simulink model "gm_uz_deadbeat_clean"  (R2022a)
settings: Solver=FixedStepDiscrete  StartTime=0.0  StopTime=1  RelTol=1e-3
libraries: hdlmdlgenlib x120, spsCurrentMeasurementLib x3, spsSeriesRLCBranchLib x2, spsDCVoltageSourceLib x1, spsPWMGenerator2LevelLib x1, spsPermanentMagnetSynchronousMachineLib x1, spsTwoLevelConverterLib x1, spsabctodq0Lib x1, spspowerguiLib x1
settings Model: Creator=go98noz  LastModifiedBy=go98noz
settings SolverCC: AlgebraicLoopSolver=TrustRegion  AutoInsertRateTranBlk=on
settings DataIOCC: LimitDataPoints=on  SaveOutput=off  SaveTime=off
settings OptimizationCC: BlockReduction=off  ConditionallyExecuteInputs=off  DefaultParameterBehavior=Inlined  InheritOutputTypeSmallerThanSingle=on  LifeSpan=inf
settings DebuggingCC: AlgebraicLoopMsg=error  InheritedTsInSrcMsg=none  SingleTaskRateTransMsg=error  UnconnectedInputMsg=warning  UnconnectedOutputMsg=warning  UnconnectedLineMsg=warning  AllowSymbolicDim=off  StrictBusMsg=ErrorOnBusTreatedAsVector  SFUnexpectedBacktrackingDiag=warning  SFNoUnconditionalDefaultTransitionDiag=warning  SFExecutionAtInitializationDiag=none  SFMachineParentedDataDiag=warning  ArithmeticOperatorsInVariantConditions=warning
settings HardwareCC: ProdBitPerPointer=32  ProdBitPerSizeT=32  ProdBitPerPtrDiffT=32  ProdLargestAtomicFloat=None  ProdIntDivRoundTo=Undefined  ProdEndianess=Unspecified  ProdWordSize=32  ProdHWDeviceType=ASIC/FPGA->ASIC/FPGA  ProdEqTarget=off
settings SFSimCC: SimUseLocalCustomCode=off  CustomCodeUndefinedFunction=UseInterfaceOnly
settings RTWCC: RTWUseLocalCustomCode=off
settings CodeAppCC: StateflowObjectComments=on
settings GRTTargetCC: TargetLangStandard=C89/C90 (ANSI)
settings ConfigComp: CovScope=ReferencedModels  CovMetricSettings=dw  CovSaveCumulativeToWorkspaceVar=on  CovSaveSingleToWorkspaceVar=on  CovExternalEMLEnable=off  CovSFcnEnable=off

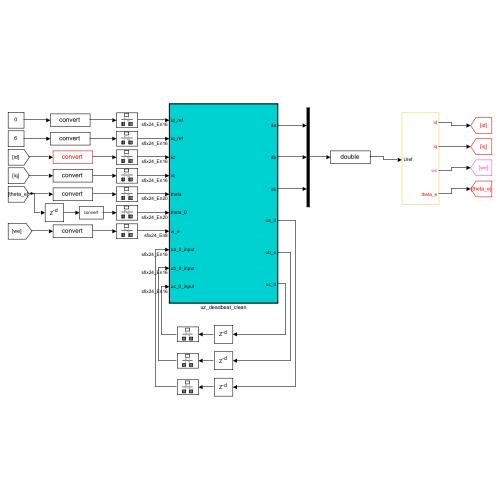
[thumbnail: Simulink's stored preview of the top-level diagram]
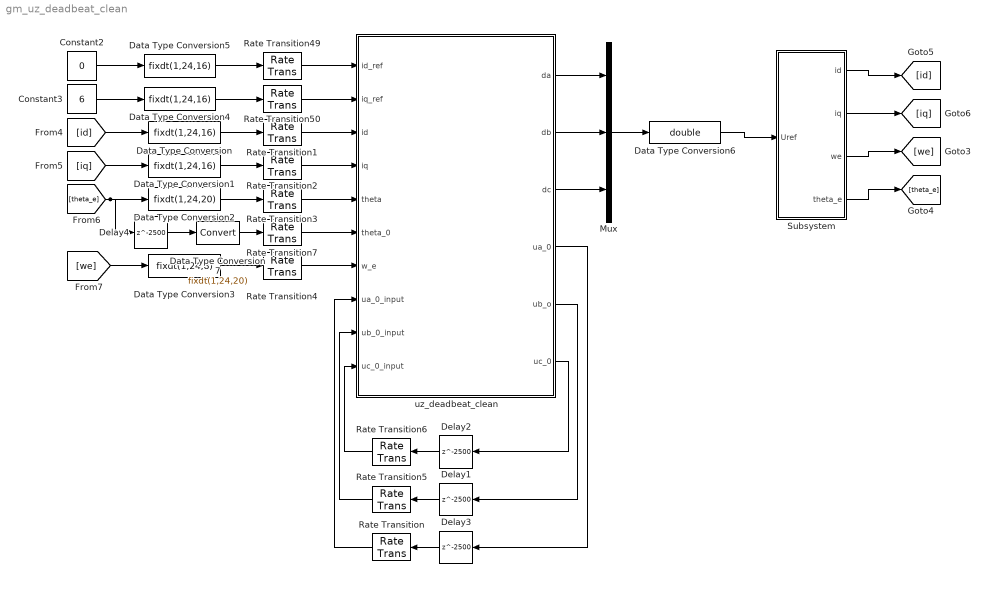
== system gm_uz_deadbeat_clean ==
  Constant2 : Constant  Value=0
  Constant3 : Constant  Value=6
  Data Type Conversion{,1,4..5} (4 alike) : DataTypeConversion  OutDataTypeStr=fixdt(1,24,16)  SaturateOnIntegerOverflow=off  RndMeth=Floor
  Data Type Conversion2 : DataTypeConversion  OutDataTypeStr=fixdt(1,24,20)  SaturateOnIntegerOverflow=off  RndMeth=Floor
  Data Type Conversion3 : DataTypeConversion  OutDataTypeStr=fixdt(1,24,8)  SaturateOnIntegerOverflow=off  RndMeth=Floor
  Data Type Conversion6 : DataTypeConversion  OutDataTypeStr=double  SaturateOnIntegerOverflow=off  RndMeth=Floor
  Data Type Conversion7 : DataTypeConversion  OutDataTypeStr=fixdt(1,24,20)  SaturateOnIntegerOverflow=off  RndMeth=Floor
  Delay{1..4} (4 alike) : Delay  DelayLength=2500  SampleTime=1e-8
  Mux : Mux  Inputs=3
  Rate Transition{,1..7,49..50} (10 alike) : RateTransition  OutPortSampleTime=1e-8
  Subsystem : Subsystem
  uz_deadbeat_clean : Subsystem  TreatAsAtomicUnit=on
  wires:
  Data Type Conversion7/1 -> Rate Transition7/1
  Rate Transition7/1 -> uz_deadbeat_clean/6(theta_0)
  Delay4/1 -> Data Type Conversion7/1
  Rate Transition/1 -> uz_deadbeat_clean/8(ua_0_input)
  Rate Transition6/1 -> uz_deadbeat_clean/10(uc_0_input)
  Rate Transition5/1 -> uz_deadbeat_clean/9(ub_0_input)
  uz_deadbeat_clean/6(uc_0) -> Delay2/1
  Delay2/1 -> Rate Transition6/1
  Delay1/1 -> Rate Transition5/1
  uz_deadbeat_clean/5(ub_o) -> Delay1/1
  Delay3/1 -> Rate Transition/1
  uz_deadbeat_clean/4(ua_0) -> Delay3/1
  Subsystem/4(theta_e) -> [theta_e]
  Subsystem/3(we) -> [we]
  Subsystem/2(iq) -> [iq]
  Subsystem/1(id) -> [id]
  Data Type Conversion6/1 -> Subsystem/1(Uref)
  uz_deadbeat_clean/3(dc) -> Mux/3
  uz_deadbeat_clean/2(db) -> Mux/2
  uz_deadbeat_clean/1(da) -> Mux/1
  Rate Transition4/1 -> uz_deadbeat_clean/7(w_e)
  [we] -> Data Type Conversion3/1
  Rate Transition3/1 -> uz_deadbeat_clean/5(theta)
  [theta_e] -> Data Type Conversion2/1, Delay4/1
  Rate Transition2/1 -> uz_deadbeat_clean/4(iq)
  [iq] -> Data Type Conversion1/1
  Rate Transition1/1 -> uz_deadbeat_clean/3(id)
  [id] -> Data Type Conversion/1
  Rate Transition50/1 -> uz_deadbeat_clean/2(iq_ref)
  Constant3/1 -> Data Type Conversion4/1
  Constant2/1 -> Data Type Conversion5/1
  Data Type Conversion2/1 -> Rate Transition3/1
  Data Type Conversion5/1 -> Rate Transition49/1
  Data Type Conversion/1 -> Rate Transition1/1
  Data Type Conversion4/1 -> Rate Transition50/1
  Data Type Conversion3/1 -> Rate Transition4/1
  Data Type Conversion1/1 -> Rate Transition2/1
  Rate Transition49/1 -> uz_deadbeat_clean/1(id_ref)
  Mux/1 -> Data Type Conversion6/1

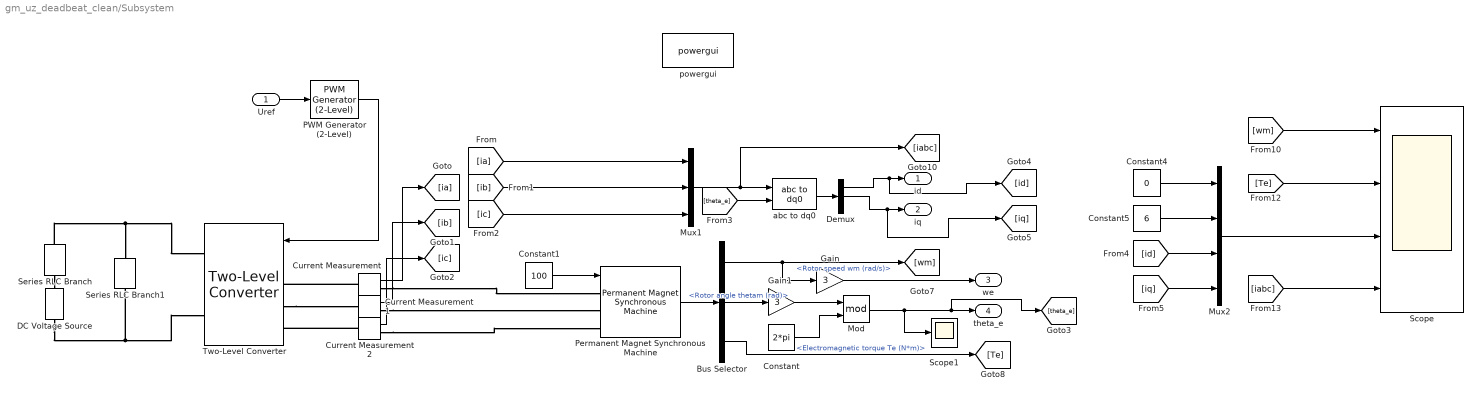
== system gm_uz_deadbeat_clean/Subsystem ==
  Uref : Inport
  Bus Selector : BusSelector  OutputSignals=Rotor speed wm (rad/s),Rotor angle thetam (rad),Electromagnetic torque Te (N*m)
  Constant : Constant  Value=2*pi
  Constant1 : Constant  Value=100
  Constant4 : Constant  Value=0
  Constant5 : Constant  Value=6
  Current Measurement : spsCurrentMeasurementLib/Current Measurement  PhasorSimulation=off  OutputType=Complex  PSBequivalent=0
  Current Measurement1 : spsCurrentMeasurementLib/Current Measurement  PhasorSimulation=off  OutputType=Complex  PSBequivalent=0
  Current Measurement2 : spsCurrentMeasurementLib/Current Measurement  PhasorSimulation=off  OutputType=Complex  PSBequivalent=0
  DC Voltage Source : spsDCVoltageSourceLib/DC Voltage Source  Amplitude=340  Measurements=None
  Demux : Demux  Outputs=3
  Gain : Gain  Gain=3
  Gain1 : Gain  Gain=3
  Mod : Math  Operator=mod
  Mux1 : Mux  Inputs=3
  Mux2 : Mux
  PWM Generator (2-Level) : spsPWMGenerator2LevelLib/PWM Generator (2-Level)  ModulatorType=Three-phase bridge (6 pulses)  ModulatorMode=Unsynchronized  Fc=20e3  Pc=0  nF=27  MinMax="[ 0  1 ]"  SamplingTechnique=Asymmetrical regular (double edge)  ModulatingSignals=off  m=0.8  Freq=60  Phase=0  Ts=1e-8  ShowCarrierOutport=off
  Permanent Magnet Synchronous Machine : spsPermanentMagnetSynchronousMachineLib/Permanent Magnet Synchronous Machine  NbPhases=3  FluxDistribution=Sinusoidal  RotorType=Round  MechanicalLoad=Speed w  PresetModel=No  ShowDetailedParameters=on  MeasurementBus=off  Resistance=1.2  Inductance=8.5e-3  dqInductances=[8.5e-3,8.5e-3]  La=0.0136  MachineConstant=Flux linkage established by magnets (V.s)  Flux=0.140  VoltageCst=76.1796  TorqueCst=0.63  Flat=120  Mechanical=[0.0002506 0.0004924 3 0]  PolePairs=3  InitialConditions=[100,0, 0,0]  InitialConditions5ph=[0 0 0 0 0 0]  RefAngle=Aligned with phase A axis (original Park)  IterativeDiscreteModel=Trapezoidal non iterative  TsBlock=-1  TsPowergui=0
  Scope : Scope  NumInputPorts=4
  Scope1 : Scope
  Series RLC Branch : spsSeriesRLCBranchLib/Series RLC Branch  LConnTagsString=__new0  RConnTagsString=__new0  BranchType=R  Resistance=1e-3  Inductance=1e-3  SetiL0=off  InitialCurrent=0  Capacitance=1e-6  Setx0=off  InitialVoltage=0  Measurements=None
  Series RLC Branch1 : spsSeriesRLCBranchLib/Series RLC Branch  LConnTagsString=__new0  RConnTagsString=__new0  BranchType=C  Resistance=1e-3  Inductance=1e-3  SetiL0=off  InitialCurrent=0  Capacitance=3300e-6  Setx0=off  InitialVoltage=0  Measurements=None
  Two-Level Converter : spsTwoLevelConverterLib/Two-Level Converter  ModelType=Switching devices  Ron=1e-3  Rs=1e6  Cs=inf  Vforward=[0,0]  Ron_Diode=1e-3  Rs_Diode=1e6  Cs_Diode=inf  Vf_Diode=1e-3  Rs_CurrentSource=inf  Ron_ACsource=1e-3
      settings: SourceProductBaseCode=PS
  abc to dq0 : spsabctodq0Lib/abc to dq0  Alignment=Aligned with phase A axis
  powergui : spspowerguiLib/powergui  Priority=1  SimulationMode=Discrete  SampleTime=1e-8  frequency=60  Iterations=50  frequencyindice=0  Pbase=100e6  ErrMax=1e-4  UnitsV=kV  UnitsW=MW  buscounter=0  FunctionMessages=off  echomessages=off  EnableUseOfTLC=off  CurrentSourceSwitches=off  DisableSnubberDevices=off  DisableRonSwitches=off  DisableVfSwitches=off  DisplayEquations=off  AutomaticDiscreteSolvers=off  SolverType=Tustin/Backward Euler (TBE)  Interpol=off  ExternalGateDelay=off  methode=off  Ts=100  x0status=blocks  SPID=on  SwTol=0  HookPort=off  NonlinearTolerance=1e-4  nMaxIteration=100  ContinueOnMaxIteration=off  RestoreLinks=warning  ResistiveCurrentMeasurement=off  Frange=[0:2:500]  Ylog=off  Xlog=on  ShowGrid=off  save=off  variable=ZData  structure=0  ZoomFFT=off  StartTime=0.0  cycles=1  DisplayStyle=1  fundamental=60  FreqAxis=off  MaxFrequency=1000  frequencyindicesteady=1  RmsSteady=1  display=off
  id : Outport
  iq : Outport  Port=2
  we : Outport  Port=3
  theta_e : Outport  Port=4
  wires:
  [ib] -> Mux1/2
  Bus Selector/3 -> [Te]  "<Electromagnetic torque Te (N*m)>"
  abc to dq0/1 -> Demux/1
  Current Measurement1/1 -> [ib]
  [wm] -> Scope/1
  [iabc] -> Scope/4
  [ia] -> Mux1/1
  [id] -> Mux2/3
  [Te] -> Scope/2
  Current Measurement/1 -> [ia]
  Constant4/1 -> Mux2/1
  Mod/1 -> Scope1/1, theta_e/1, [theta_e]
  Uref/1 -> PWM Generator (2-Level)/1
  Permanent Magnet Synchronous Machine/1 -> Bus Selector/1
  Gain1/1 -> Mod/1
  [ic] -> Mux1/3
  Demux/2 -> iq/1, [iq]
  Demux/1 -> id/1, [id]
  Bus Selector/1 -> [wm], Gain/1  "<Rotor speed wm (rad/s)>"
  Bus Selector/2 -> Gain1/1  "<Rotor angle thetam (rad)>"
  [theta_e] -> abc to dq0/2
  Mux1/1 -> abc to dq0/1, [iabc]
  Gain/1 -> we/1
  Mux2/1 -> Scope/3
  Constant5/1 -> Mux2/2
  [iq] -> Mux2/4
  Current Measurement2/1 -> [ic]
  Constant1/1 -> Permanent Magnet Synchronous Machine/1
  PWM Generator (2-Level)/1 -> Two-Level Converter/1
  Constant/1 -> Mod/2
  connections:
  Current Measurement/RConn1 -- Permanent Magnet Synchronous Machine/LConn1
  Current Measurement2/LConn1 -- Two-Level Converter/LConn3
  Two-Level Converter/LConn2 -- Current Measurement1/LConn1
  Series RLC Branch/LConn1 -- Series RLC Branch1/LConn1 -- Two-Level Converter/RConn1
  Current Measurement1/RConn1 -- Permanent Magnet Synchronous Machine/LConn2
  Series RLC Branch/RConn1 -- DC Voltage Source/RConn1
  Current Measurement2/RConn1 -- Permanent Magnet Synchronous Machine/LConn3
  Current Measurement/LConn1 -- Two-Level Converter/LConn1
  DC Voltage Source/LConn1 -- Two-Level Converter/RConn2 -- Series RLC Branch1/RConn1

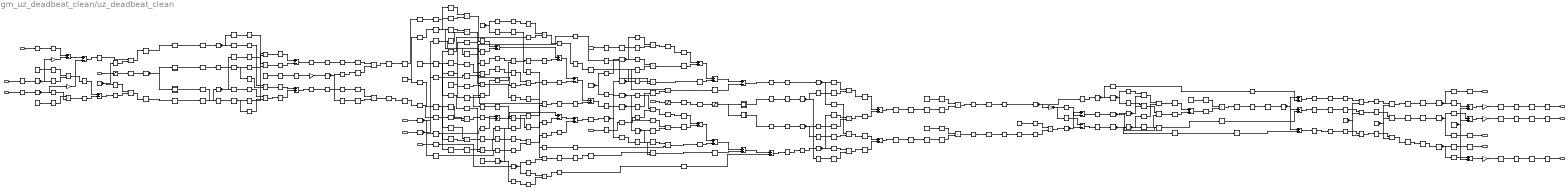
== system gm_uz_deadbeat_clean/uz_deadbeat_clean ==
  id_ref : Inport  OutDataTypeStr=fixdt(1, 24, 16)  PortDimensions=1  SampleTime=1e-08
  iq_ref : Inport  Port=2  OutDataTypeStr=fixdt(1, 24, 16)  PortDimensions=1  SampleTime=1e-08
  id : Inport  Port=3  OutDataTypeStr=fixdt(1, 24, 16)  PortDimensions=1  SampleTime=1e-08
  iq : Inport  Port=4  OutDataTypeStr=fixdt(1, 24, 16)  PortDimensions=1  SampleTime=1e-08
  theta : Inport  Port=5  OutDataTypeStr=fixdt(1, 24, 20)  PortDimensions=1  SampleTime=1e-08
  theta_0 : Inport  Port=6  OutDataTypeStr=fixdt(1, 24, 20)  PortDimensions=1  SampleTime=1e-08
  w_e : Inport  Port=7  OutDataTypeStr=fixdt(1, 24, 8)  PortDimensions=1  SampleTime=1e-08
  ua_0_input : Inport  Port=8  OutDataTypeStr=fixdt(1, 24, 16)  PortDimensions=1  SampleTime=1e-08
  ub_0_input : Inport  Port=9  OutDataTypeStr=fixdt(1, 24, 16)  PortDimensions=1  SampleTime=1e-08
  uc_0_input : Inport  Port=10  OutDataTypeStr=fixdt(1, 24, 16)  PortDimensions=1  SampleTime=1e-08
  Add1 : Sum  Inputs=+-  AccumDataTypeStr=fixdt(1, 49, 39)  OutDataTypeStr=fixdt(1, 49, 39)  SampleTime=1e-08
  Add10 : Sum  Inputs=+-  AccumDataTypeStr=fixdt(1, 49, 24)  OutDataTypeStr=fixdt(1, 49, 24)  SampleTime=1e-08
  Add11 : Sum  AccumDataTypeStr=fixdt(1, 49, 24)  OutDataTypeStr=fixdt(1, 49, 24)  SampleTime=1e-08
  Add12 : Sum  Inputs=+-  AccumDataTypeStr=fixdt(1, 49, 39)  OutDataTypeStr=fixdt(1, 49, 39)  SampleTime=1e-08
  Add13 : Sum  Inputs=--  AccumDataTypeStr=fixdt(1, 50, 39)  OutDataTypeStr=fixdt(1, 50, 39)  SampleTime=1e-08
  Add{14..20} (7 alike) : Sum  AccumDataTypeStr=fixdt(1, 25, 16)  OutDataTypeStr=fixdt(1, 25, 16)  SampleTime=1e-08
  Add2 : Sum  AccumDataTypeStr=fixdt(1, 49, 32)  OutDataTypeStr=fixdt(1, 49, 32)  SampleTime=1e-08
  Add3 : Sum  Inputs=+-  AccumDataTypeStr=fixdt(1, 49, 32)  OutDataTypeStr=fixdt(1, 49, 32)  SampleTime=1e-08
  Add4_stage2 : Sum  AccumDataTypeStr=fixdt(1, 83, 56)  OutDataTypeStr=fixdt(1, 49, 30)  SampleTime=1e-08
  Add4_stage3 : Sum  Inputs=+-  AccumDataTypeStr=fixdt(1, 83, 56)  OutDataTypeStr=fixdt(1, 83, 56)  SampleTime=1e-08
  Add4_stage4 : Sum  AccumDataTypeStr=fixdt(1, 83, 56)  OutDataTypeStr=fixdt(1, 83, 56)  SampleTime=1e-08
  Add5_stage2 : Sum  AccumDataTypeStr=fixdt(1, 83, 56)  OutDataTypeStr=fixdt(1, 49, 30)  SampleTime=1e-08
  Add5_stage3 : Sum  Inputs=+-  AccumDataTypeStr=fixdt(1, 83, 56)  OutDataTypeStr=fixdt(1, 83, 56)  SampleTime=1e-08
  Add5_stage4 : Sum  Inputs=+-  AccumDataTypeStr=fixdt(1, 83, 56)  OutDataTypeStr=fixdt(1, 83, 56)  SampleTime=1e-08
  Add5_stage5 : Sum  Inputs=+-  AccumDataTypeStr=fixdt(1, 83, 56)  OutDataTypeStr=fixdt(1, 83, 56)  SampleTime=1e-08
  Add7_stage2 : Sum  Inputs=+-  AccumDataTypeStr=fixdt(1, 73, 44)  OutDataTypeStr=fixdt(1, 73, 44)  SampleTime=1e-08
  Add7_stage3 : Sum  AccumDataTypeStr=fixdt(1, 73, 44)  OutDataTypeStr=fixdt(1, 74, 44)  SampleTime=1e-08
  Add7_stage4 : Sum  Inputs=+-  AccumDataTypeStr=fixdt(1, 73, 44)  OutDataTypeStr=fixdt(1, 73, 44)  SampleTime=1e-08
  Add8_stage2 : Sum  Inputs=+-  AccumDataTypeStr=fixdt(1, 73, 44)  OutDataTypeStr=fixdt(1, 73, 44)  SampleTime=1e-08
  Add8_stage3 : Sum  AccumDataTypeStr=fixdt(1, 73, 44)  OutDataTypeStr=fixdt(1, 74, 44)  SampleTime=1e-08
  Add8_stage4 : Sum  AccumDataTypeStr=fixdt(1, 73, 44)  OutDataTypeStr=fixdt(1, 75, 44)  SampleTime=1e-08
  Add8_stage5 : Sum  AccumDataTypeStr=fixdt(1, 73, 44)  OutDataTypeStr=fixdt(1, 73, 44)  SampleTime=1e-08
  Add_stage2 : Sum  Inputs=+-  AccumDataTypeStr=fixdt(1, 50, 39)  OutDataTypeStr=fixdt(1, 50, 39)  SampleTime=1e-08
  Add_stage3 : Sum  Inputs=+-  AccumDataTypeStr=fixdt(1, 50, 39)  OutDataTypeStr=fixdt(1, 50, 39)  SampleTime=1e-08
  Constant : Constant  Value=0.6666717529296875  OutDataTypeStr=fixdt(1, 24, 16)  SampleTime=1e-08
  Constant1 : Constant  Value=2.50004231929779052734375e-05  OutDataTypeStr=fixdt(0, 32, 30)  SampleTime=1e-08
  Constant10 : Constant  Value=0.001838207244873046875  OutDataTypeStr=fixdt(0, 24, 22)  SampleTime=1e-08
  Constant12 : Constant  Value=544  OutDataTypeStr=fixdt(0, 24, 8)  SampleTime=1e-08
  Constant2 : Constant  Value=1.200000762939453125  OutDataTypeStr=fixdt(1, 24, 18)  SampleTime=1e-08
  Constant3 : Constant  Value=0.01360034942626953125  OutDataTypeStr=fixdt(0, 24, 20)  SampleTime=1e-08
  Constant5 : Constant  Value=0.1400001049041748046875  OutDataTypeStr=fixdt(0, 24, 22)  SampleTime=1e-08
  Constant6 : Constant  Value=340  OutDataTypeStr=fixdt(0, 24, 8)  SampleTime=1e-08
  Constant7 : Constant  Value=-1  OutDataTypeStr=fixdt(1, 24, 16)  SampleTime=1e-08
  Constant8 : Constant  OutDataTypeStr=fixdt(1, 24, 16)  SampleTime=1e-08
  Constant9 : Constant  OutDataTypeStr=fixdt(1, 24, 16)  SampleTime=1e-08
  Data Type Conversion{6..11,14..15,22..38} (25 alike) : DataTypeConversion  OutDataTypeStr=fixdt(1, 24, 16)  SampleTime=1e-08  SaturateOnIntegerOverflow=off  RndMeth=Floor
  Data Type Conversion{12..13,17..18,20..21} (6 alike) : DataTypeConversion  OutDataTypeStr=fixdt(1, 24, 8)  SampleTime=1e-08  SaturateOnIntegerOverflow=off  RndMeth=Floor
  Data Type Conversion48 : DataTypeConversion  OutDataTypeStr=fixdt(0, 24, 8)  SampleTime=1e-08  SaturateOnIntegerOverflow=off  RndMeth=Floor
  From{,1..21,24..30,36..41,44..50,54..60,62..80,82} (69 alike) : hdlmdlgenlib/Buffer
      settings: SourceProductBaseCode=SL
  From_outbuff_out_pipe : Delay  DelayLength=double(10)  InitialCondition=0  SampleTime=1e-08
  Gain : Product  Inputs=**  OutDataTypeStr=fixdt(1, 48, 38)  SampleTime=1e-08
  Gain1 : Gain  Gain="fi(0,1,24,23,\"hex\",\"400000\")"  ParamDataTypeStr=fixdt(1, 24, 23)  OutDataTypeStr=fixdt(1, 48, 39)  SampleTime=1e-08
  Gain10 : Gain  Gain="fi(0,1,25,24,\"hex\",\"0800000\")"  ParamDataTypeStr=fixdt(1, 25, 24)  OutDataTypeStr=fixdt(1, 50, 40)  SampleTime=1e-08
  Gain11 : Gain  Gain="fi(0,1,25,24,\"hex\",\"0800000\")"  ParamDataTypeStr=fixdt(1, 25, 24)  OutDataTypeStr=fixdt(1, 50, 40)  SampleTime=1e-08
  Gain12 : Product  Inputs=**  OutDataTypeStr=fixdt(1, 48, 38)  SampleTime=1e-08
  Gain12_const : Constant  Value=0.00588000006973743438720703125  OutDataTypeStr=fixdt(1, 24, 30)  SampleTime=1e-08
  Gain2 : Gain  Gain="fi(0,1,24,23,\"hex\",\"400000\")"  ParamDataTypeStr=fixdt(1, 24, 23)  OutDataTypeStr=fixdt(1, 48, 39)  SampleTime=1e-08
  Gain3 : Product  Inputs=**  OutDataTypeStr=fixdt(1, 48, 39)  SampleTime=1e-08
  Gain3_const : Constant  Value=0.866025447845458984375  OutDataTypeStr=fixdt(1, 24, 23)  SampleTime=1e-08
  Gain4 : Product  Inputs=**  OutDataTypeStr=fixdt(1, 48, 39)  SampleTime=1e-08
  Gain4_const : Constant  Value=0.866025447845458984375  OutDataTypeStr=fixdt(1, 24, 23)  SampleTime=1e-08
  Gain5 : Gain  Gain="fi(0,1,24,23,\"hex\",\"400000\")"  ParamDataTypeStr=fixdt(1, 24, 23)  OutDataTypeStr=fixdt(1, 48, 39)  SampleTime=1e-08
  Gain6 : Product  Inputs=**  OutDataTypeStr=fixdt(1, 48, 39)  SampleTime=1e-08
  Gain6_const : Constant  Value=0.86600005626678466796875  OutDataTypeStr=fixdt(1, 24, 23)  SampleTime=1e-08
  Gain7 : Product  Inputs=**  OutDataTypeStr=fixdt(1, 50, 41)  SampleTime=1e-08
  Gain7_const : Constant  Value=-0.5  OutDataTypeStr=fixdt(1, 25, 25)  SampleTime=1e-08
  Gain8 : Gain  Gain="fi(0,0,24,24,\"hex\",\"800000\")"  ParamDataTypeStr=fixdt(0, 24, 24)  OutDataTypeStr=fixdt(0, 48, 32)  SampleTime=1e-08
  Gain9 : Gain  Gain="fi(0,1,25,24,\"hex\",\"0800000\")"  ParamDataTypeStr=fixdt(1, 25, 24)  OutDataTypeStr=fixdt(1, 50, 40)  SampleTime=1e-08
  Gain_const : Constant  Value=0.00588000006973743438720703125  OutDataTypeStr=fixdt(1, 24, 30)  SampleTime=1e-08
  Goto{,1..22,24..25,27..52} (51 alike) : hdlmdlgenlib/Buffer
      settings: SourceProductBaseCode=SL
  HwModeRegister{,1..81} (82 alike) : Delay  DelayLength=double(1)  InitialCondition=0  SampleTime=1e-08
  Min1_stage1 : MinMax  Function=max  Inputs=2
  Min1_stage2 : MinMax  Function=max  Inputs=2
  Min2_stage1 : MinMax  Function=max  Inputs=2
  Min3_stage1 : MinMax  Function=max  Inputs=2
  Min4_stage1 : MinMax  Function=max  Inputs=2
  Min5_stage1 : MinMax  Inputs=2
  Min6_stage1 : MinMax  Inputs=2
  Min7_stage1 : MinMax  Inputs=2
  Min_stage1 : MinMax  Inputs=2
  Min_stage2 : MinMax  Inputs=2
  PipelineRegister{,1..40} (41 alike) : Delay  DelayLength=double(1)  InitialCondition=0  SampleTime=1e-08
  Product : Product  Inputs=**  OutDataTypeStr=fixdt(1, 74, 55)  SampleTime=1e-08
  Product1 : Product  Inputs=**  OutDataTypeStr=fixdt(1, 73, 55)  SampleTime=1e-08
  Product11 : Product  Inputs=**  OutDataTypeStr=fixdt(1, 72, 52)  SampleTime=1e-08
  Product12 : Product  Inputs=**  OutDataTypeStr=fixdt(1, 72, 44)  SampleTime=1e-08
  Product{14..15,18..19,24..29} (10 alike) : Product  Inputs=**  OutDataTypeStr=fixdt(1, 48, 24)  SampleTime=1e-08
  Product16 : Product  Inputs=**  OutDataTypeStr=fixdt(1, 48, 34)  SampleTime=1e-08
  Product17 : Product  Inputs=**  OutDataTypeStr=fixdt(1, 72, 44)  SampleTime=1e-08
  Product{2..5} (4 alike) : Product  Inputs=**  OutDataTypeStr=fixdt(1, 48, 32)  SampleTime=1e-08
  Product20 : Product  Inputs=**  OutDataTypeStr=fixdt(1, 48, 34)  SampleTime=1e-08
  Product{6,9,22,36} (4 alike) : Product  Inputs=**  OutDataTypeStr=fixdt(1, 48, 30)  SampleTime=1e-08
  Product30 : Product  Inputs=**  OutDataTypeStr=fixdt(1, 72, 56)  SampleTime=1e-08
  Product31 : Product  Inputs=**  OutDataTypeStr=fixdt(1, 80, 54)  SampleTime=1e-08
  Product32 : Product  Inputs=**  OutDataTypeStr=fixdt(1, 72, 56)  SampleTime=1e-08
  Product33 : Product  Inputs=**  OutDataTypeStr=fixdt(1, 80, 54)  SampleTime=1e-08
  Product34 : Product  Inputs=**  OutDataTypeStr=fixdt(1, 48, 38)  SampleTime=1e-08
  Product35 : Product  Inputs=**  OutDataTypeStr=fixdt(1, 56, 38)  SampleTime=1e-08
  Product37 : Product  Inputs=**  OutDataTypeStr=fixdt(1, 48, 28)  SampleTime=1e-08
  Product38 : Product  Inputs=**  OutDataTypeStr=fixdt(1, 48, 28)  SampleTime=1e-08
  Product7 : Product  Inputs=**  OutDataTypeStr=fixdt(1, 48, 38)  SampleTime=1e-08
  Product8 : Product  Inputs=**  OutDataTypeStr=fixdt(1, 56, 38)  SampleTime=1e-08
  Saturation : Saturate  UpperLimit="fi(0,1,24,20,\"hex\",\"64872b\")"  LowerLimit="fi(0,1,24,20,\"hex\",\"000000\")"  SampleTime=1e-08  OutDataTypeStr=fixdt(1, 24, 20)
  Saturation1 : Saturate  UpperLimit="fi(0,1,24,20,\"hex\",\"64872b\")"  LowerLimit="fi(0,1,24,20,\"hex\",\"000000\")"  SampleTime=1e-08  OutDataTypeStr=fixdt(1, 24, 20)
  Saturation2 : Saturate  UpperLimit="fi(0,1,24,20,\"hex\",\"64872b\")"  LowerLimit="fi(0,1,24,20,\"hex\",\"000000\")"  SampleTime=1e-08  OutDataTypeStr=fixdt(1, 24, 20)
  Trigonometric Function : Subsystem
  Trigonometric Function1 : Subsystem
  Trigonometric Function2 : Subsystem
  Trigonometric Function3 : Subsystem
  delayMatch{,9,31..35} (7 alike) : Delay  DelayLength=double(10)  InitialCondition=0  SampleTime=1e-08
  delayMatch{1,8,17,21..23} (6 alike) : Delay  DelayLength=double(8)  InitialCondition=0  SampleTime=1e-08
  delayMatch{2,4,6,10,12,14..15} (7 alike) : Delay  DelayLength=double(14)  InitialCondition=0  SampleTime=1e-08
  delayMatch{3,7,11,18,20} (5 alike) : Delay  DelayLength=double(18)  InitialCondition=0  SampleTime=1e-08
  delayMatch{5,13,24..27,29..30} (8 alike) : Delay  DelayLength=double(2)  InitialCondition=0  SampleTime=1e-08
  delayMatch16 : Delay  DelayLength=double(16)  InitialCondition=0  SampleTime=1e-08
  delayMatch19 : Delay  DelayLength=double(16)  InitialCondition=0  SampleTime=1e-08
  delayMatch28 : Delay  DelayLength=double(4)  InitialCondition=0  SampleTime=1e-08
  dtc{,1..9} (10 alike) : DataTypeConversion  OutDataTypeStr=fixdt(1, 24, 16)  SampleTime=1e-08  SaturateOnIntegerOverflow=off  RndMeth=Floor
  da : Outport  SampleTime=1e-08  VectorParamsAs1DForOutWhenUnconnected=off
  db : Outport  Port=2  SampleTime=1e-08  VectorParamsAs1DForOutWhenUnconnected=off
  dc : Outport  Port=3  SampleTime=1e-08  VectorParamsAs1DForOutWhenUnconnected=off
  ua_0 : Outport  Port=4  SampleTime=1e-08  VectorParamsAs1DForOutWhenUnconnected=off
  ub_o : Outport  Port=5  SampleTime=1e-08  VectorParamsAs1DForOutWhenUnconnected=off
  uc_0 : Outport  Port=6  SampleTime=1e-08  VectorParamsAs1DForOutWhenUnconnected=off
  wires:
  id_ref/1 -> Goto5/1
  iq_ref/1 -> Goto6/1
  id/1 -> Goto7/1
  iq/1 -> Goto8/1
  theta/1 -> Saturation/1
  theta_0/1 -> Saturation2/1
  w_e/1 -> Goto10/1
  ua_0_input/1 -> Goto/1
  ub_0_input/1 -> Goto1/1
  uc_0_input/1 -> Goto2/1
  Add_stage3/1 -> HwModeRegister/1
  Add1/1 -> HwModeRegister3/1
  Add10/1 -> Data Type Conversion20/1
  Add11/1 -> Data Type Conversion21/1
  Add12/1 -> Data Type Conversion25/1
  Add13/1 -> Data Type Conversion26/1
  Add14/1 -> HwModeRegister81/1
  Add15/1 -> Data Type Conversion30/1
  Add16/1 -> Data Type Conversion31/1
  Add17/1 -> Data Type Conversion32/1
  Add18/1 -> Gain9/1
  Add19/1 -> Gain10/1
  Add2/1 -> Data Type Conversion8/1
  Add20/1 -> Gain11/1
  Add3/1 -> Data Type Conversion9/1
  Add4_stage4/1 -> Data Type Conversion14/1
  Add5_stage5/1 -> Data Type Conversion15/1
  Add7_stage4/1 -> Data Type Conversion17/1
  Add8_stage5/1 -> Data Type Conversion18/1
  Constant/1 -> HwModeRegister1/1, HwModeRegister2/1
  Constant1/1 -> Goto15/1
  Constant10/1 -> Goto50/1, Goto49/1
  Constant12/1 -> Goto52/1, Goto51/1
  Constant2/1 -> Goto16/1
  Constant3/1 -> Goto18/1, Goto17/1
  Constant5/1 -> Goto19/1
  Constant6/1 -> Goto20/1
  Constant7/1 -> Min2_stage1/2, Min3_stage1/2, Min4_stage1/2
  Constant8/1 -> Min5_stage1/2, Min6_stage1/2, Min7_stage1/2
  Constant9/1 -> Add20/2, Add19/2, Add18/2
  Data Type Conversion10/1 -> Goto11/1
  Data Type Conversion11/1 -> Goto12/1
  Data Type Conversion12/1 -> Goto37/1
  Data Type Conversion13/1 -> Goto38/1
  Data Type Conversion14/1 -> Goto21/1
  Data Type Conversion15/1 -> Goto22/1
  Data Type Conversion17/1 -> Goto24/1
  Data Type Conversion18/1 -> Goto25/1
  Data Type Conversion20/1 -> Goto29/1
  Data Type Conversion21/1 -> Goto30/1
  Data Type Conversion22/1 -> Goto31/1
  Data Type Conversion23/1 -> Goto32/1
  Data Type Conversion24/1 -> Goto33/1
  Data Type Conversion25/1 -> Goto34/1
  Data Type Conversion26/1 -> Goto35/1
  Data Type Conversion27/1 -> Goto27/1
  Data Type Conversion28/1 -> Goto28/1
  Data Type Conversion29/1 -> Goto36/1
  Data Type Conversion30/1 -> Goto39/1
  Data Type Conversion31/1 -> Goto40/1
  Data Type Conversion32/1 -> Goto41/1
  Data Type Conversion33/1 -> Goto44/1
  Data Type Conversion34/1 -> Goto43/1
  Data Type Conversion35/1 -> Goto42/1
  Data Type Conversion36/1 -> Goto45/1
  Data Type Conversion37/1 -> Goto46/1
  Data Type Conversion38/1 -> Goto47/1
  delayMatch2/1 -> HwModeRegister35/1
  Data Type Conversion6/1 -> Goto3/1
  Data Type Conversion7/1 -> Goto4/1
  Data Type Conversion8/1 -> Goto13/1
  Data Type Conversion9/1 -> Goto14/1
  From_outbuff_out_pipe/1 -> da/1
  delayMatch31/1 -> db/1
  delayMatch1/1 -> HwModeRegister38/1
  From11/1 -> HwModeRegister62/1, HwModeRegister64/1
  From12/1 -> HwModeRegister21/1, HwModeRegister61/1
  From13/1 -> HwModeRegister39/1, HwModeRegister59/1
  From14/1 -> HwModeRegister8/1, HwModeRegister10/1
  From15/1 -> HwModeRegister16/1, HwModeRegister18/1
  From16/1 -> HwModeRegister63/1
  delayMatch3/1 -> Add4_stage2/2
  From18/1 -> HwModeRegister41/1
  From19/1 -> HwModeRegister66/1
  delayMatch32/1 -> dc/1
  From20/1 -> HwModeRegister67/1
  delayMatch5/1 -> HwModeRegister43/1
  From24/1 -> HwModeRegister69/1
  delayMatch11/1 -> Add5_stage2/2
  From26/1 -> HwModeRegister45/1
  From27/1 -> HwModeRegister50/1, HwModeRegister53/1
  From28/1 -> HwModeRegister51/1
  delayMatch13/1 -> HwModeRegister47/1
  delayMatch33/1 -> ua_0/1
  From30/1 -> HwModeRegister5/1
  From36/1 -> HwModeRegister9/1
  From37/1 -> HwModeRegister11/1, HwModeRegister12/1
  From38/1 -> HwModeRegister13/1
  From39/1 -> HwModeRegister56/1
  delayMatch34/1 -> ub_o/1
  From40/1 -> HwModeRegister57/1
  From41/1 -> HwModeRegister7/1
  From44/1 -> HwModeRegister17/1
  From45/1 -> HwModeRegister19/1, HwModeRegister22/1
  From46/1 -> HwModeRegister23/1
  From47/1 -> HwModeRegister54/1
  From48/1 -> HwModeRegister24/1, HwModeRegister55/1
  From49/1 -> HwModeRegister15/1
  delayMatch35/1 -> uc_0/1
  From50/1 -> HwModeRegister25/1
  From54/1 -> HwModeRegister48/1, HwModeRegister52/1, HwModeRegister68/1
  From55/1 -> HwModeRegister26/1, HwModeRegister30/1
  From56/1 -> HwModeRegister28/1, HwModeRegister32/1
  delayMatch17/1 -> HwModeRegister27/1
  delayMatch21/1 -> HwModeRegister29/1
  From59/1 -> HwModeRegister71/1
  From6/1 -> Add_stage2/1
  From60/1 -> HwModeRegister73/1
  From62/1 -> Data Type Conversion24/1, Gain5/1
  From63/1 -> HwModeRegister79/1
  delayMatch25/1 -> Min_stage1/1
  From65/1 -> Min_stage1/2, Min1_stage1/2
  From66/1 -> dtc/1, dtc2/1
  From67/1 -> HwModeRegister34/1
  From68/1 -> HwModeRegister36/1
  From69/1 -> Gain8/1
  From7/1 -> Gain1/1, HwModeRegister75/1
  From70/1 -> Add17/1, Add16/1, Add15/1
  delayMatch28/1 -> Add15/2
  delayMatch29/1 -> Add16/2
  delayMatch30/1 -> Add17/2
  From74/1 -> Min2_stage1/1
  From75/1 -> Min3_stage1/1
  From76/1 -> Min4_stage1/1
  From77/1 -> Add18/1
  From78/1 -> Add19/1
  From79/1 -> Add20/1
  From8/1 -> Gain2/1, HwModeRegister77/1
  From80/1 -> Saturation1/1
  From82/1 -> Trigonometric Function/1(In1), Trigonometric Function1/1(In1)
  delayMatch/1 -> HwModeRegister20/1
  PipelineRegister35/1 -> Data Type Conversion22/1
  Gain1/1 -> Add_stage2/2
  Gain10/1 -> Data Type Conversion37/1
  Gain11/1 -> Data Type Conversion38/1
  PipelineRegister36/1 -> Data Type Conversion23/1
  Gain2/1 -> Add_stage3/2
  PipelineRegister37/1 -> Add1/1
  PipelineRegister38/1 -> Add1/2
  delayMatch24/1 -> Add12/2
  PipelineRegister39/1 -> Add13/2, Add12/1
  PipelineRegister40/1 -> Data Type Conversion29/1
  Gain8/1 -> Data Type Conversion48/1
  Gain9/1 -> Data Type Conversion36/1
  dtc1/1 -> Add14/1
  dtc3/1 -> Add14/2
  dtc4/1 -> Min5_stage1/1
  dtc5/1 -> Min6_stage1/1
  dtc6/1 -> Min7_stage1/1
  dtc7/1 -> Data Type Conversion33/1
  dtc8/1 -> Data Type Conversion34/1
  dtc9/1 -> Data Type Conversion35/1
  PipelineRegister/1 -> Data Type Conversion6/1
  PipelineRegister1/1 -> Data Type Conversion7/1
  delayMatch15/1 -> Add5_stage5/2
  PipelineRegister3/1 -> Add7_stage4/2
  delayMatch7/1 -> Add7_stage2/1
  PipelineRegister5/1 -> Add7_stage2/2
  PipelineRegister6/1 -> Add7_stage3/2
  PipelineRegister7/1 -> Add8_stage4/2
  delayMatch18/1 -> Add8_stage2/1
  PipelineRegister9/1 -> Add8_stage2/2
  PipelineRegister10/1 -> Add2/1
  PipelineRegister11/1 -> Add8_stage3/2
  delayMatch20/1 -> Add8_stage5/2
  PipelineRegister13/1 -> Add10/1
  PipelineRegister14/1 -> Add10/2
  PipelineRegister15/1 -> Add11/1
  PipelineRegister16/1 -> Add11/2
  PipelineRegister17/1 -> Data Type Conversion12/1
  PipelineRegister18/1 -> Data Type Conversion13/1
  PipelineRegister19/1 -> Add2/2
  delayMatch4/1 -> Add4_stage3/2
  delayMatch6/1 -> Add4_stage4/2
  delayMatch12/1 -> Add5_stage3/2
  delayMatch14/1 -> Add5_stage4/2
  PipelineRegister24/1 -> HwModeRegister44/1
  PipelineRegister25/1 -> HwModeRegister46/1
  PipelineRegister26/1 -> HwModeRegister4/1
  delayMatch19/1 -> HwModeRegister14/1
  delayMatch16/1 -> HwModeRegister6/1
  PipelineRegister29/1 -> Add3/2
  PipelineRegister30/1 -> Add3/1
  PipelineRegister31/1 -> Add4_stage2/1
  PipelineRegister32/1 -> HwModeRegister40/1
  PipelineRegister33/1 -> HwModeRegister42/1
  PipelineRegister34/1 -> Add5_stage2/1
  Saturation/1 -> Goto9/1
  Saturation1/1 -> Trigonometric Function2/1(In1), Trigonometric Function3/1(In1)
  Saturation2/1 -> Goto48/1
  Trigonometric Function/1(Out1) -> Data Type Conversion11/1
  Trigonometric Function1/1(Out1) -> Data Type Conversion10/1
  Trigonometric Function2/1(Out1) -> Data Type Conversion28/1
  Trigonometric Function3/1(Out1) -> Data Type Conversion27/1
  From/1 -> From_outbuff_out_pipe/1
  Goto45/1 -> From/1
  Goto46/1 -> From1/1
  Goto4/1 -> From10/1
  Goto49/1 -> From11/1
  Goto11/1 -> From12/1
  Goto12/1 -> From13/1
  Goto51/1 -> From14/1
  Goto52/1 -> From15/1
  Goto37/1 -> From16/1
  Goto7/1 -> From29/1, From17/1
  Goto16/1 -> From46/1, From38/1, From26/1, From18/1
  Goto10/1 -> From48/1, From40/1, From27/1, From19/1
  Goto47/1 -> From2/1
  Goto15/1 -> From28/1, From20/1
  Goto8/1 -> From25/1, From21/1
  Goto38/1 -> From24/1
  Goto44/1 -> From77/1, From3/1
  Goto19/1 -> From50/1, From30/1
  Goto9/1 -> From80/1
  Goto5/1 -> From36/1
  Goto21/1 -> From49/1, From37/1
  Goto18/1 -> From39/1
  Goto43/1 -> From78/1, From4/1
  Goto22/1 -> From45/1, From41/1
  Goto6/1 -> From44/1
  Goto17/1 -> From47/1
  Goto42/1 -> From79/1, From5/1
  Goto50/1 -> From54/1
  Goto24/1 -> From55/1
  Goto25/1 -> From56/1
  Goto27/1 -> From57/1
  Goto28/1 -> From58/1
  Goto29/1 -> From59/1
  Goto/1 -> From6/1
  Goto30/1 -> From60/1
  Goto31/1 -> From62/1
  Goto32/1 -> From63/1
  Goto33/1 -> From71/1, From64/1
  Goto34/1 -> From72/1, From65/1
  Goto35/1 -> From73/1, From66/1
  Goto13/1 -> From67/1
  Goto14/1 -> From68/1
  Goto20/1 -> From69/1
  Goto1/1 -> From7/1
  Goto36/1 -> From70/1
  Goto39/1 -> From74/1
  Goto40/1 -> From75/1
  Goto41/1 -> From76/1
  Goto2/1 -> From8/1
  Goto48/1 -> From82/1
  Goto3/1 -> From9/1
  Add_stage2/1 -> Add_stage3/1
  Add4_stage2/1 -> Add4_stage3/1
  Add4_stage3/1 -> Add4_stage4/1
  Add5_stage2/1 -> Add5_stage3/1
  Add5_stage3/1 -> Add5_stage4/1
  Add5_stage4/1 -> Add5_stage5/1
  Add7_stage2/1 -> Add7_stage3/1
  Add7_stage3/1 -> Add7_stage4/1
  Add8_stage2/1 -> Add8_stage3/1
  Add8_stage3/1 -> Add8_stage4/1
  Add8_stage4/1 -> Add8_stage5/1
  Min_stage1/1 -> Min_stage2/1
  dtc/1 -> Min_stage2/2
  Min_stage2/1 -> dtc1/1
  Min1_stage1/1 -> Min1_stage2/1
  dtc2/1 -> Min1_stage2/2
  Min1_stage2/1 -> dtc3/1
  Min2_stage1/1 -> dtc4/1
  Min3_stage1/1 -> dtc5/1
  Min4_stage1/1 -> dtc6/1
  Min5_stage1/1 -> dtc7/1
  Min6_stage1/1 -> dtc8/1
  Min7_stage1/1 -> dtc9/1
  Gain_const/1 -> HwModeRegister70/1
  Gain12_const/1 -> HwModeRegister72/1
  Gain3_const/1 -> HwModeRegister74/1
  Gain4_const/1 -> HwModeRegister76/1
  Gain6_const/1 -> HwModeRegister78/1
  Gain7_const/1 -> HwModeRegister80/1
  delayMatch9/1 -> HwModeRegister58/1
  delayMatch8/1 -> HwModeRegister60/1
  delayMatch10/1 -> HwModeRegister37/1
  From17/1 -> delayMatch3/1, HwModeRegister65/1
  PipelineRegister20/1 -> delayMatch4/1
  From21/1 -> delayMatch5/1
  PipelineRegister21/1 -> delayMatch6/1
  PipelineRegister4/1 -> delayMatch7/1
  From10/1 -> delayMatch8/1, delayMatch1/1
  From9/1 -> delayMatch9/1, delayMatch/1
  Data Type Conversion48/1 -> delayMatch10/1, delayMatch2/1
  From25/1 -> delayMatch11/1, HwModeRegister49/1
  PipelineRegister22/1 -> delayMatch12/1
  From29/1 -> delayMatch13/1
  PipelineRegister23/1 -> delayMatch14/1
  PipelineRegister2/1 -> delayMatch15/1
  PipelineRegister28/1 -> delayMatch16/1
  delayMatch23/1 -> HwModeRegister33/1
  PipelineRegister8/1 -> delayMatch18/1
  PipelineRegister27/1 -> delayMatch19/1
  PipelineRegister12/1 -> delayMatch20/1
  delayMatch22/1 -> HwModeRegister31/1
  From58/1 -> delayMatch22/1, delayMatch21/1
  From57/1 -> delayMatch23/1, delayMatch17/1
  delayMatch26/1 -> Add13/1
  delayMatch27/1 -> Min1_stage1/1
  Gain5/1 -> delayMatch26/1, delayMatch24/1
  From64/1 -> delayMatch27/1, delayMatch25/1
  From71/1 -> delayMatch28/1
  From72/1 -> delayMatch29/1
  From73/1 -> delayMatch30/1
  From1/1 -> delayMatch31/1
  From2/1 -> delayMatch32/1
  From3/1 -> delayMatch33/1
  From4/1 -> delayMatch34/1
  From5/1 -> delayMatch35/1
  Product/1 -> PipelineRegister/1
  HwModeRegister/1 -> Product/1
  HwModeRegister1/1 -> Product/2
  Product1/1 -> PipelineRegister1/1
  HwModeRegister2/1 -> Product1/1
  HwModeRegister3/1 -> Product1/2
  Product11/1 -> PipelineRegister2/1
  HwModeRegister4/1 -> Product11/1
  HwModeRegister5/1 -> Product11/2
  Product12/1 -> PipelineRegister3/1
  HwModeRegister6/1 -> Product12/1
  HwModeRegister7/1 -> Product12/2
  Product14/1 -> PipelineRegister4/1
  HwModeRegister8/1 -> Product14/1
  HwModeRegister9/1 -> Product14/2
  Product15/1 -> PipelineRegister5/1
  HwModeRegister10/1 -> Product15/1
  HwModeRegister11/1 -> Product15/2
  Product16/1 -> PipelineRegister6/1
  HwModeRegister12/1 -> Product16/1
  HwModeRegister13/1 -> Product16/2
  Product17/1 -> PipelineRegister7/1
  HwModeRegister14/1 -> Product17/1
  HwModeRegister15/1 -> Product17/2
  Product18/1 -> PipelineRegister8/1
  HwModeRegister16/1 -> Product18/1
  HwModeRegister17/1 -> Product18/2
  Product19/1 -> PipelineRegister9/1
  HwModeRegister18/1 -> Product19/1
  HwModeRegister19/1 -> Product19/2
  Product2/1 -> PipelineRegister10/1
  HwModeRegister20/1 -> Product2/1
  HwModeRegister21/1 -> Product2/2
  Product20/1 -> PipelineRegister11/1
  HwModeRegister22/1 -> Product20/1
  HwModeRegister23/1 -> Product20/2
  Product22/1 -> PipelineRegister12/1
  HwModeRegister24/1 -> Product22/1
  HwModeRegister25/1 -> Product22/2
  Product24/1 -> PipelineRegister13/1
  HwModeRegister26/1 -> Product24/1
  HwModeRegister27/1 -> Product24/2
  Product25/1 -> PipelineRegister14/1
  HwModeRegister28/1 -> Product25/1
  HwModeRegister29/1 -> Product25/2
  Product26/1 -> PipelineRegister15/1
  HwModeRegister30/1 -> Product26/1
  HwModeRegister31/1 -> Product26/2
  Product27/1 -> PipelineRegister16/1
  HwModeRegister32/1 -> Product27/1
  HwModeRegister33/1 -> Product27/2
  Product28/1 -> PipelineRegister17/1
  HwModeRegister34/1 -> Product28/1
  HwModeRegister35/1 -> Product28/2
  Product29/1 -> PipelineRegister18/1
  HwModeRegister36/1 -> Product29/1
  HwModeRegister37/1 -> Product29/2
  Product3/1 -> PipelineRegister19/1
  HwModeRegister38/1 -> Product3/1
  HwModeRegister39/1 -> Product3/2
  Product30/1 -> PipelineRegister20/1
  HwModeRegister40/1 -> Product30/1
  HwModeRegister41/1 -> Product30/2
  Product31/1 -> PipelineRegister21/1
  HwModeRegister42/1 -> Product31/1
  HwModeRegister43/1 -> Product31/2
  Product32/1 -> PipelineRegister22/1
  HwModeRegister44/1 -> Product32/1
  HwModeRegister45/1 -> Product32/2
  Product33/1 -> PipelineRegister23/1
  HwModeRegister46/1 -> Product33/1
  HwModeRegister47/1 -> Product33/2
  Product34/1 -> PipelineRegister24/1
  HwModeRegister48/1 -> Product34/1
  HwModeRegister49/1 -> Product34/2
  Product35/1 -> PipelineRegister25/1
  HwModeRegister50/1 -> Product35/1
  HwModeRegister51/1 -> Product35/2
  Product36/1 -> PipelineRegister26/1
  HwModeRegister52/1 -> Product36/1
  HwModeRegister53/1 -> Product36/2
  Product37/1 -> PipelineRegister27/1
  HwModeRegister54/1 -> Product37/1
  HwModeRegister55/1 -> Product37/2
  Product38/1 -> PipelineRegister28/1
  HwModeRegister56/1 -> Product38/1
  HwModeRegister57/1 -> Product38/2
  Product4/1 -> PipelineRegister29/1
  HwModeRegister58/1 -> Product4/1
  HwModeRegister59/1 -> Product4/2
  Product5/1 -> PipelineRegister30/1
  HwModeRegister60/1 -> Product5/1
  HwModeRegister61/1 -> Product5/2
  Product6/1 -> PipelineRegister31/1
  HwModeRegister62/1 -> Product6/1
  HwModeRegister63/1 -> Product6/2
  Product7/1 -> PipelineRegister32/1
  HwModeRegister64/1 -> Product7/1
  HwModeRegister65/1 -> Product7/2
  Product8/1 -> PipelineRegister33/1
  HwModeRegister66/1 -> Product8/1
  HwModeRegister67/1 -> Product8/2
  Product9/1 -> PipelineRegister34/1
  HwModeRegister68/1 -> Product9/1
  HwModeRegister69/1 -> Product9/2
  Gain/1 -> PipelineRegister35/1
  HwModeRegister70/1 -> Gain/1
  HwModeRegister71/1 -> Gain/2
  Gain12/1 -> PipelineRegister36/1
  HwModeRegister72/1 -> Gain12/1
  HwModeRegister73/1 -> Gain12/2
  Gain3/1 -> PipelineRegister37/1
  HwModeRegister74/1 -> Gain3/1
  HwModeRegister75/1 -> Gain3/2
  Gain4/1 -> PipelineRegister38/1
  HwModeRegister76/1 -> Gain4/1
  HwModeRegister77/1 -> Gain4/2
  Gain6/1 -> PipelineRegister39/1
  HwModeRegister78/1 -> Gain6/1
  HwModeRegister79/1 -> Gain6/2
  Gain7/1 -> PipelineRegister40/1
  HwModeRegister80/1 -> Gain7/1
  HwModeRegister81/1 -> Gain7/2

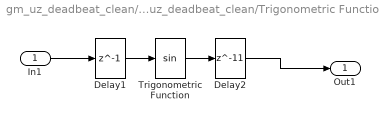
== system gm_uz_deadbeat_clean/uz_deadbeat_clean/Trigonometric Function ==
  In1 : Inport
  Delay1 : Delay  DelayLength=1
  Delay2 : Delay  DelayLength=11
  Trigonometric Function : Trigonometry  ApproximationMethod=CORDIC
  Out1 : Outport
  wires:
  In1/1 -> Delay1/1
  Delay1/1 -> Trigonometric Function/1
  Trigonometric Function/1 -> Delay2/1
  Delay2/1 -> Out1/1

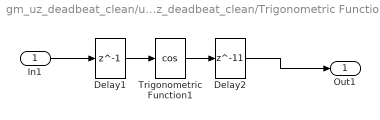
== system gm_uz_deadbeat_clean/uz_deadbeat_clean/Trigonometric Function1 ==
  In1 : Inport
  Delay1 : Delay  DelayLength=1
  Delay2 : Delay  DelayLength=11
  Trigonometric Function1 : Trigonometry  Operator=cos  ApproximationMethod=CORDIC
  Out1 : Outport
  wires:
  In1/1 -> Delay1/1
  Delay1/1 -> Trigonometric Function1/1
  Trigonometric Function1/1 -> Delay2/1
  Delay2/1 -> Out1/1

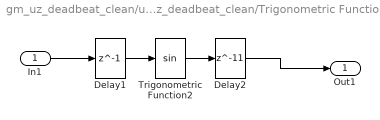
== system gm_uz_deadbeat_clean/uz_deadbeat_clean/Trigonometric Function2 ==
  In1 : Inport
  Delay1 : Delay  DelayLength=1
  Delay2 : Delay  DelayLength=11
  Trigonometric Function2 : Trigonometry  ApproximationMethod=CORDIC
  Out1 : Outport
  wires:
  In1/1 -> Delay1/1
  Delay1/1 -> Trigonometric Function2/1
  Trigonometric Function2/1 -> Delay2/1
  Delay2/1 -> Out1/1

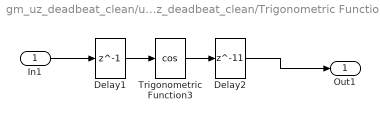
== system gm_uz_deadbeat_clean/uz_deadbeat_clean/Trigonometric Function3 ==
  In1 : Inport
  Delay1 : Delay  DelayLength=1
  Delay2 : Delay  DelayLength=11
  Trigonometric Function3 : Trigonometry  Operator=cos  ApproximationMethod=CORDIC
  Out1 : Outport
  wires:
  In1/1 -> Delay1/1
  Delay1/1 -> Trigonometric Function3/1
  Trigonometric Function3/1 -> Delay2/1
  Delay2/1 -> Out1/1
